simulink model "mimo3"  (R2021b)
settings: Solver=VariableStepAuto  StartTime=0.0  StopTime=10.0  RelTol=1e-3
libraries: cstblocks x5
settings Model: Creator=Hu  LastModifiedBy=Hu

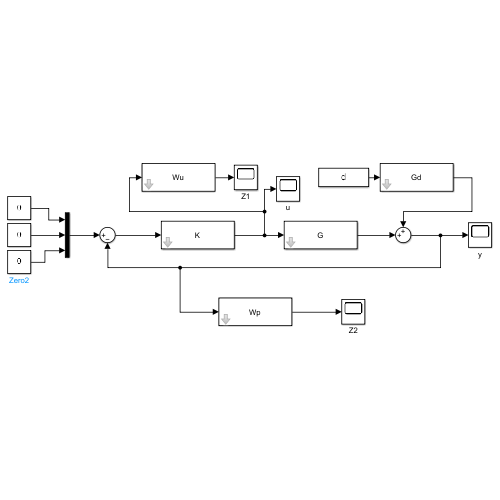
[thumbnail: Simulink's stored preview of the top-level diagram]
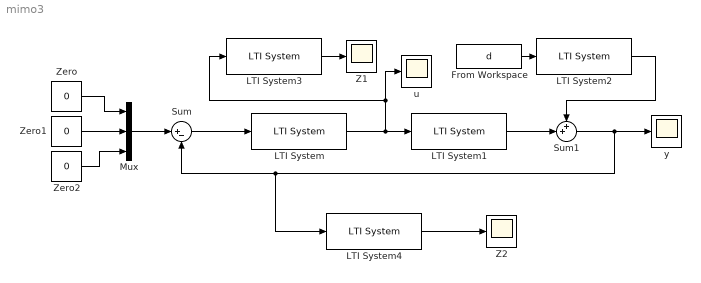
== system mimo3 ==
  From Workspace : FromWorkspace  VariableName=d
  LTI System : cstblocks/LTI System  sys=K  IC=[]
  LTI System1 : cstblocks/LTI System  sys=G  IC=[]
  LTI System2 : cstblocks/LTI System  sys=Gd  IC=[]
  LTI System3 : cstblocks/LTI System  sys=Wu  IC=[]
  LTI System4 : cstblocks/LTI System  sys=Wp  IC=[]
  Mux : Mux  Inputs=3
  Sum : Sum  Inputs=|+-
  Sum1 : Sum  Inputs=++|
  Z1 : Scope
  Z2 : Scope
  Zero : Constant  Value=0  OutDataTypeStr=Inherit: Inherit via back propagation
  Zero1 : Constant  Value=0  OutDataTypeStr=Inherit: Inherit via back propagation
  Zero2 : Constant  Value=0  OutDataTypeStr=Inherit: Inherit via back propagation
  u : Scope
  y : Scope
  wires:
  Sum/1 -> LTI System/1
  LTI System/1 -> u/1, LTI System3/1, LTI System1/1
  LTI System1/1 -> Sum1/2
  LTI System2/1 -> Sum1/1
  Sum1/1 -> LTI System4/1, Sum/2, y/1
  LTI System4/1 -> Z2/1
  LTI System3/1 -> Z1/1
  From Workspace/1 -> LTI System2/1
  Mux/1 -> Sum/1
  Zero2/1 -> Mux/3
  Zero1/1 -> Mux/2
  Zero/1 -> Mux/1
